simulink model "CerebellumIODCNAbstractFext"  (Simulink 7.4)
settings: Solver=ode3  StartTime=0.0  StopTime=1.  FixedStep=0.002  RelTol=1e-3
values from neighbouring files (symbols this model uses):
  RRedKuKa = RRedKuKa    [LaunchCerebellumSimulink.m]    (also in LaunchCerebellumSimulinkExternalForce.m; MANIPULATORS.mat = )
undefined symbols (not defined in the file or in its folder): frne
libraries: simulink x1
(part 2 of 2)

== system CerebellumIODCNAbstractFext/Subsystem/Subsystem IO1/IO Subsystem /bloque1 IO3 ==
  Time Firing Poisson : Inport  OutDataType=sfix(16)  OutScaling=2^0
  TimefiringIO0 : Outport  OutDataType=sfix(16)  OutScaling=2^0
  TimefiringIO1 : Outport  Port=2  OutDataType=sfix(16)  OutScaling=2^0
  TimefiringIO2 : Outport  Port=3  OutDataType=sfix(16)  OutScaling=2^0
  TimefiringIO3 : Outport  Port=4  OutDataType=sfix(16)  OutScaling=2^0
  TimefiringIO4 : Outport  Port=5  OutDataType=sfix(16)  OutScaling=2^0
  TimefiringIO5 : Outport  Port=6  OutDataType=sfix(16)  OutScaling=2^0
  TimefiringIO6 : Outport  Port=7  OutDataType=sfix(16)  OutScaling=2^0
  TimefiringIO7 : Outport  Port=8  OutDataType=sfix(16)  OutScaling=2^0
  wires:
  Time Firing Poisson/1 -> TimefiringIO0/1, TimefiringIO1/1, TimefiringIO2/1, TimefiringIO3/1, TimefiringIO4/1, TimefiringIO5/1, TimefiringIO6/1, TimefiringIO7/1

== system CerebellumIODCNAbstractFext/Subsystem/Subsystem IO1/IO Subsystem /bloque1 IO4 ==
  Time Firing Poisson : Inport  OutDataType=sfix(16)  OutScaling=2^0
  TimefiringIO0 : Outport  OutDataType=sfix(16)  OutScaling=2^0
  TimefiringIO1 : Outport  Port=2  OutDataType=sfix(16)  OutScaling=2^0
  TimefiringIO2 : Outport  Port=3  OutDataType=sfix(16)  OutScaling=2^0
  TimefiringIO3 : Outport  Port=4  OutDataType=sfix(16)  OutScaling=2^0
  TimefiringIO4 : Outport  Port=5  OutDataType=sfix(16)  OutScaling=2^0
  TimefiringIO5 : Outport  Port=6  OutDataType=sfix(16)  OutScaling=2^0
  TimefiringIO6 : Outport  Port=7  OutDataType=sfix(16)  OutScaling=2^0
  TimefiringIO7 : Outport  Port=8  OutDataType=sfix(16)  OutScaling=2^0
  wires:
  Time Firing Poisson/1 -> TimefiringIO0/1, TimefiringIO1/1, TimefiringIO2/1, TimefiringIO3/1, TimefiringIO4/1, TimefiringIO5/1, TimefiringIO6/1, TimefiringIO7/1

== system CerebellumIODCNAbstractFext/Subsystem/Subsystem IO1/IO Subsystem /bloque1 IO5 ==
  Time Firing Poisson : Inport  OutDataType=sfix(16)  OutScaling=2^0
  TimefiringIO0 : Outport  OutDataType=sfix(16)  OutScaling=2^0
  TimefiringIO1 : Outport  Port=2  OutDataType=sfix(16)  OutScaling=2^0
  TimefiringIO2 : Outport  Port=3  OutDataType=sfix(16)  OutScaling=2^0
  TimefiringIO3 : Outport  Port=4  OutDataType=sfix(16)  OutScaling=2^0
  TimefiringIO4 : Outport  Port=5  OutDataType=sfix(16)  OutScaling=2^0
  TimefiringIO5 : Outport  Port=6  OutDataType=sfix(16)  OutScaling=2^0
  TimefiringIO6 : Outport  Port=7  OutDataType=sfix(16)  OutScaling=2^0
  TimefiringIO7 : Outport  Port=8  OutDataType=sfix(16)  OutScaling=2^0
  wires:
  Time Firing Poisson/1 -> TimefiringIO0/1, TimefiringIO1/1, TimefiringIO2/1, TimefiringIO3/1, TimefiringIO4/1, TimefiringIO5/1, TimefiringIO6/1, TimefiringIO7/1

== system CerebellumIODCNAbstractFext/Subsystem/Subsystem IO1/IO Subsystem /Poisson1 IO/IO-FIRE ==
  Random[a b] & I : Inport  OutDataType=sfix(16)  OutScaling=2^0
  Constant : Constant  OutDataTypeMode=boolean  OutDataType=fixdt(1, 16)  OutScaling=2^0  OutDataTypeStr=boolean
  Constant1 : Constant  Value=0  OutDataTypeMode=boolean  OutDataType=fixdt(1, 16)  OutScaling=2^0  OutDataTypeStr=boolean
  Switch3 : Switch  Criteria=u2 > Threshold
  Time Firing : Outport  OutDataType=sfix(16)  OutScaling=2^0
  wires:
  Switch3/1 -> Time Firing/1
  Random[a b] & I/1 -> Switch3/2
  Constant1/1 -> Switch3/3
  Constant/1 -> Switch3/1

== system CerebellumIODCNAbstractFext/Subsystem/Subsystem IO1/IO Subsystem /Poisson1 IO/IO-FIRE2 ==
  Random[a b] & I : Inport  OutDataType=sfix(16)  OutScaling=2^0
  Constant : Constant  OutDataTypeMode=boolean  OutDataType=fixdt(1, 16)  OutScaling=2^0  OutDataTypeStr=boolean
  Constant1 : Constant  Value=0  OutDataTypeMode=boolean  OutDataType=fixdt(1, 16)  OutScaling=2^0  OutDataTypeStr=boolean
  Switch3 : Switch  Criteria=u2 > Threshold
  Time Firing : Outport  OutDataType=sfix(16)  OutScaling=2^0
  wires:
  Switch3/1 -> Time Firing/1
  Random[a b] & I/1 -> Switch3/2
  Constant1/1 -> Switch3/3
  Constant/1 -> Switch3/1

== system CerebellumIODCNAbstractFext/Subsystem/Subsystem IO1/IO Subsystem /Poisson1 IO/Subsystem ==
  Par max : Inport  OutDataType=sfix(16)  OutScaling=2^0
  error : Inport  Port=2  OutDataType=sfix(16)  OutScaling=2^0
  Mux2 : Mux  Inputs=2
  S-Function : S-Function  FunctionName=errormanagementmod  EnableBusSupport=off
  I : Outport  OutDataType=sfix(16)  OutScaling=2^0
  wires:
  Par max/1 -> Mux2/1
  error/1 -> Mux2/2
  S-Function/1 -> I/1
  Mux2/1 -> S-Function/1

== system CerebellumIODCNAbstractFext/Subsystem/Subsystem IO1/IO Subsystem /Poisson1 IO/interval[a b] ==
  Mux5 : Mux  Inputs=2
  a : Constant  Value=a  OutDataType=sfix(16)  OutScaling=2^0
  b : Constant  Value=b  OutDataType=sfix(16)  OutScaling=2^0
  I : Outport  OutDataType=sfix(16)  OutScaling=2^0
  wires:
  a/1 -> Mux5/1
  b/1 -> Mux5/2
  Mux5/1 -> I/1

== system CerebellumIODCNAbstractFext/Subsystem/Subsystem IO1/IO Subsystem /Poisson1 IO1/IO-FIRE ==
  Random[a b] & I : Inport  OutDataType=sfix(16)  OutScaling=2^0
  Constant : Constant  OutDataTypeMode=boolean  OutDataType=fixdt(1, 16)  OutScaling=2^0  OutDataTypeStr=boolean
  Constant1 : Constant  Value=0  OutDataTypeMode=boolean  OutDataType=fixdt(1, 16)  OutScaling=2^0  OutDataTypeStr=boolean
  Switch3 : Switch  Criteria=u2 > Threshold
  Time Firing : Outport  OutDataType=sfix(16)  OutScaling=2^0
  wires:
  Switch3/1 -> Time Firing/1
  Random[a b] & I/1 -> Switch3/2
  Constant1/1 -> Switch3/3
  Constant/1 -> Switch3/1

== system CerebellumIODCNAbstractFext/Subsystem/Subsystem IO1/IO Subsystem /Poisson1 IO1/IO-FIRE2 ==
  Random[a b] & I : Inport  OutDataType=sfix(16)  OutScaling=2^0
  Constant : Constant  OutDataTypeMode=boolean  OutDataType=fixdt(1, 16)  OutScaling=2^0  OutDataTypeStr=boolean
  Constant1 : Constant  Value=0  OutDataTypeMode=boolean  OutDataType=fixdt(1, 16)  OutScaling=2^0  OutDataTypeStr=boolean
  Switch3 : Switch  Criteria=u2 > Threshold
  Time Firing : Outport  OutDataType=sfix(16)  OutScaling=2^0
  wires:
  Switch3/1 -> Time Firing/1
  Random[a b] & I/1 -> Switch3/2
  Constant1/1 -> Switch3/3
  Constant/1 -> Switch3/1

== system CerebellumIODCNAbstractFext/Subsystem/Subsystem IO1/IO Subsystem /Poisson1 IO1/Subsystem ==
  Par max : Inport  OutDataType=sfix(16)  OutScaling=2^0
  error : Inport  Port=2  OutDataType=sfix(16)  OutScaling=2^0
  Mux2 : Mux  Inputs=2
  S-Function : S-Function  FunctionName=errormanagementmod  EnableBusSupport=off
  I : Outport  OutDataType=sfix(16)  OutScaling=2^0
  wires:
  Par max/1 -> Mux2/1
  error/1 -> Mux2/2
  S-Function/1 -> I/1
  Mux2/1 -> S-Function/1

== system CerebellumIODCNAbstractFext/Subsystem/Subsystem IO1/IO Subsystem /Poisson1 IO1/interval[a b] ==
  Mux5 : Mux  Inputs=2
  a : Constant  Value=a  OutDataType=sfix(16)  OutScaling=2^0
  b : Constant  Value=b  OutDataType=sfix(16)  OutScaling=2^0
  I : Outport  OutDataType=sfix(16)  OutScaling=2^0
  wires:
  a/1 -> Mux5/1
  b/1 -> Mux5/2
  Mux5/1 -> I/1

== system CerebellumIODCNAbstractFext/Subsystem/Subsystem IO1/IO Subsystem /Poisson1 IO2/IO-FIRE ==
  Random[a b] & I : Inport  OutDataType=sfix(16)  OutScaling=2^0
  Constant : Constant  OutDataTypeMode=boolean  OutDataType=fixdt(1, 16)  OutScaling=2^0  OutDataTypeStr=boolean
  Constant1 : Constant  Value=0  OutDataTypeMode=boolean  OutDataType=fixdt(1, 16)  OutScaling=2^0  OutDataTypeStr=boolean
  Switch3 : Switch  Criteria=u2 > Threshold
  Time Firing : Outport  OutDataType=sfix(16)  OutScaling=2^0
  wires:
  Switch3/1 -> Time Firing/1
  Random[a b] & I/1 -> Switch3/2
  Constant1/1 -> Switch3/3
  Constant/1 -> Switch3/1

== system CerebellumIODCNAbstractFext/Subsystem/Subsystem IO1/IO Subsystem /Poisson1 IO2/IO-FIRE2 ==
  Random[a b] & I : Inport  OutDataType=sfix(16)  OutScaling=2^0
  Constant : Constant  OutDataTypeMode=boolean  OutDataType=fixdt(1, 16)  OutScaling=2^0  OutDataTypeStr=boolean
  Constant1 : Constant  Value=0  OutDataTypeMode=boolean  OutDataType=fixdt(1, 16)  OutScaling=2^0  OutDataTypeStr=boolean
  Switch3 : Switch  Criteria=u2 > Threshold
  Time Firing : Outport  OutDataType=sfix(16)  OutScaling=2^0
  wires:
  Switch3/1 -> Time Firing/1
  Random[a b] & I/1 -> Switch3/2
  Constant1/1 -> Switch3/3
  Constant/1 -> Switch3/1

== system CerebellumIODCNAbstractFext/Subsystem/Subsystem IO1/IO Subsystem /Poisson1 IO2/Subsystem ==
  Par max : Inport  OutDataType=sfix(16)  OutScaling=2^0
  error : Inport  Port=2  OutDataType=sfix(16)  OutScaling=2^0
  Mux2 : Mux  Inputs=2
  S-Function : S-Function  FunctionName=errormanagementmod  EnableBusSupport=off
  I : Outport  OutDataType=sfix(16)  OutScaling=2^0
  wires:
  Par max/1 -> Mux2/1
  error/1 -> Mux2/2
  S-Function/1 -> I/1
  Mux2/1 -> S-Function/1

== system CerebellumIODCNAbstractFext/Subsystem/Subsystem IO1/IO Subsystem /Poisson1 IO2/interval[a b] ==
  Mux5 : Mux  Inputs=2
  a : Constant  Value=a  OutDataType=sfix(16)  OutScaling=2^0
  b : Constant  Value=b  OutDataType=sfix(16)  OutScaling=2^0
  I : Outport  OutDataType=sfix(16)  OutScaling=2^0
  wires:
  a/1 -> Mux5/1
  b/1 -> Mux5/2
  Mux5/1 -> I/1
